simulink model "asg3_2_nonlinear"  (R2020b)
settings: Solver=VariableStepAuto  StartTime=0.0  StopTime=10.0  RelTol=1e-3
settings Model: Creator=Master  LastModifiedBy=Pratyush Jaiswal
settings DebuggingCC: SFMachineParentedDataDiag=error

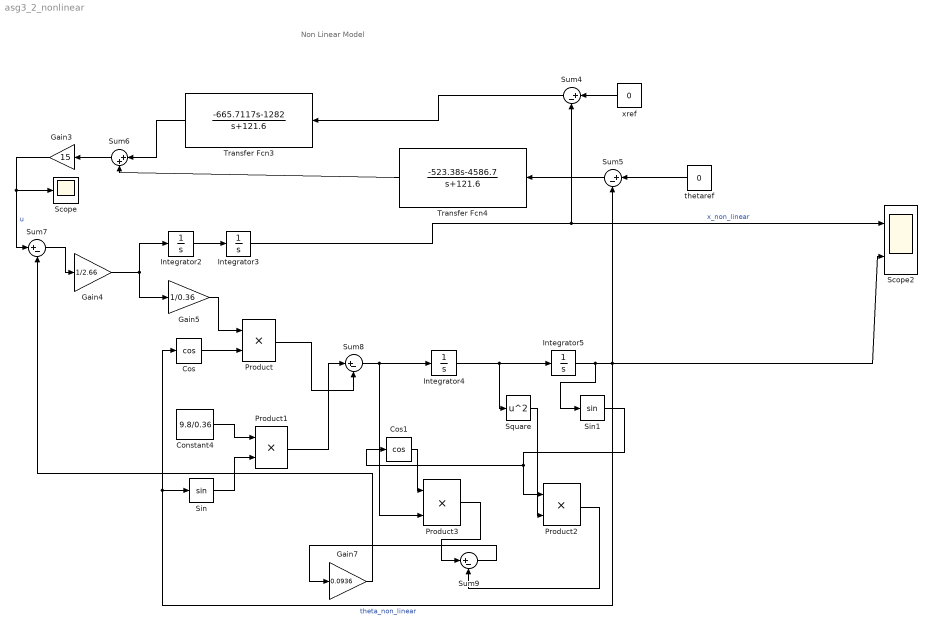
== system asg3_2_nonlinear ==
  note: Non Linear Model
  Constant4 : Constant  Value=9.8/0.36
  Cos : Trigonometry  Operator=cos
  Cos1 : Trigonometry  Operator=cos
  Gain3 : Gain  Gain=15
  Gain4 : Gain  Gain=1/2.66
  Gain5 : Gain  Gain=1/0.36
  Gain7 : Gain  Gain=0.0936
  Integrator2 : Integrator
  Integrator3 : Integrator
  Integrator4 : Integrator
  Integrator5 : Integrator  InitialCondition=0.15
  Product{,1..3} (4 alike) : Product
  Scope : Scope
  Scope2 : Scope  NumInputPorts=2
  Sin : Trigonometry
  Sin1 : Trigonometry
  Square : Math  Operator=square  SaturateOnIntegerOverflow=on
  Sum{4..5,7..9} (5 alike) : Sum  Inputs=|+-
  Sum6 : Sum  Inputs=|++
  Transfer Fcn3 : TransferFcn  Numerator=[-665.7117 -1282]  Denominator=[1 121.6]
  Transfer Fcn4 : TransferFcn  Numerator=[-523.38 -4586.7]  Denominator=[1 121.6]
  thetaref : Constant  Value=0
  xref : Constant  Value=0
  wires:
  Product/1 -> Sum8/2
  Sin/1 -> Product1/2
  Constant4/1 -> Product1/1
  Sum7/1 -> Gain4/1
  Gain5/1 -> Product/1
  Gain4/1 -> Integrator2/1, Gain5/1
  Sum6/1 -> Gain3/1
  Gain3/1 -> Scope/1, Sum7/1  "u"
  Transfer Fcn4/1 -> Sum6/2
  Transfer Fcn3/1 -> Sum6/1
  Sum4/1 -> Transfer Fcn3/1
  Integrator3/1 -> Scope2/1, Sum4/2  "x_non_linear"
  Gain7/1 -> Sum7/2
  thetaref/1 -> Sum5/1
  Integrator4/1 -> Square/1, Integrator5/1
  Sum9/1 -> Gain7/1
  Sum8/1 -> Product3/2, Integrator4/1
  Sum5/1 -> Transfer Fcn4/1
  xref/1 -> Sum4/1
  Integrator2/1 -> Integrator3/1
  Product1/1 -> Sum8/1
  Product2/1 -> Sum9/2
  Cos/1 -> Product/2
  Cos1/1 -> Product3/1
  Sin1/1 -> Cos1/1, Product2/1
  Product3/1 -> Sum9/1
  Square/1 -> Product2/2
  Integrator5/1 -> Sum5/2, Scope2/2, Sin/1, Cos/1, Sin1/1  "theta_non_linear"
